simulink model "chap1_1"  (Simulink 8.8)
settings: Solver=VariableStepAuto  StartTime=0.0  StopTime=10.0  RelTol=1e-3
settings Model: SuppressorTable=22 serialization::archive 11 0 3 0 0 0 0 0  Creator=guoshaopan  LastModifiedBy=guoshaopan
settings DataIOCC: LimitDataPoints=off  SaveFormat=Dataset  SignalLoggingSaveFormat=Dataset
settings OptimizationCC: LifeSpan=auto
settings DebuggingCC: UnderspecifiedInitializationDetection=Simplified  MergeDetectMultiDrivingBlocksExec=error  FcnCallInpInsideContextMsg=error  StateNameClashWarn=none  SFUnexpectedBacktrackingDiag=error  SFNoUnconditionalDefaultTransitionDiag=error  SFExecutionAtInitializationDiag=warning
settings HardwareCC: ProdBitPerPointer=64  ProdBitPerSizeT=64  ProdBitPerPtrDiffT=64  ProdLargestAtomicFloat=Float  ProdIntDivRoundTo=Zero  ProdEndianess=LittleEndian  ProdWordSize=64  ProdHWDeviceType=Intel->x86-64 (Windows64)
settings ModelReferenceCC: PropagateSignalLabelsOutOfModel=on
settings GRTTargetCC: TargetLangStandard=C99 (ISO)  GeneratePreprocessorConditionals=Use local settings  CombineOutputUpdateFcns=on  GRTInterface=off
settings ConfigComp: CovMetricSettings=dwe  CovHtmlReporting=off  CovSaveCumulativeToWorkspaceVar=off  CovSaveSingleToWorkspaceVar=off  CovExternalEMLEnable=on

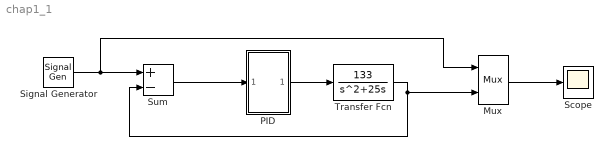
== system chap1_1 ==
  Mux : Mux  Inputs=2
  PID : Subsystem
  Scope : Scope
  Signal Generator : SignalGenerator  Frequency=0.20
  Sum : Sum  Inputs=+-
  Transfer Fcn : TransferFcn  Numerator=[133]  Denominator=[1 25 0]
  wires:
  Signal Generator/1 -> Mux/1, Sum/1
  Sum/1 -> PID/1(In1)
  PID/1(Out1) -> Transfer Fcn/1
  Transfer Fcn/1 -> Mux/2, Sum/2
  Mux/1 -> Scope/1

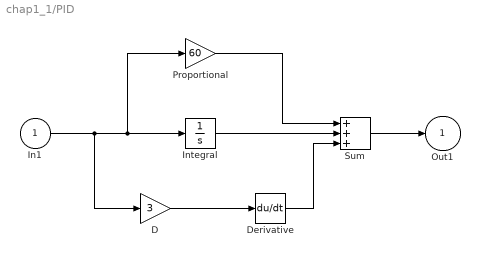
== system chap1_1/PID ==
  In1 : Inport
  D : Gain  Gain=3
  Derivative : Derivative
  Integral : Integrator
  Proportional : Gain  Gain=60
  Sum : Sum  Inputs=+++
  Out1 : Outport
  wires:
  Proportional/1 -> Sum/1
  Integral/1 -> Sum/2
  In1/1 -> D/1, Proportional/1, Integral/1
  D/1 -> Derivative/1
  Derivative/1 -> Sum/3
  Sum/1 -> Out1/1
